simulink model "elec_switching_power_supply"  (R2016a)
settings: Solver=ode23t  StartTime=0.0  StopTime=0.006  RelTol=1e-3
PostLoadFcn:
  | controller_choice=1; % Variant selection variable
InitFcn:
  | if ~exist('T_junction1','var')
  |   T_junction1 = 404.79;
  | end
  | if ~exist('T_junction2','var')
  |   T_junction2 = 384.83;
  | end
libraries: fl_lib x11, elec_lib x7, nesl_utility x3, simulink x1
CloseFcn:
  | try close(h1_elec_switching_power_supply), end
  | try close(h2_elec_switching_power_supply), end
  | try clear elec_sps_log tout controller_choice, end
Description:
  | Synchronous Buck Converter
  | 
  | This example shows how to model a switching power supply that converts a 30V DC
  | supply into a regulated 15V DC supply. The model can be used to both size the
  | inductance L and smoothing capacitor C, as well as to design the feedback
  | controller. By selecting between continuous, discrete and fixed-point controllers, the
  | impact of discretization and using limited numerical precision can be explored.
  | 
  | Modeling the switching devices as MOSFETs rather than ideal switches ensures that
  | device on-resistances are correctly represented. The model also captures the
  | switch-on/switch-off timing of the devices, this depending primarily on the gate
  | capacitance values and the PWM driver output resistance.
  | 
  | If you have Simscape(TM) Power Systems(TM), see example model
  | power_switching_power_supply for an abstracted version of this model that
  | uses ideal switching to give faster simulation times. The model here can be used to
  | determine the on-resistance values required for the ideal switches, plus timing
  | offsets if necessary. Using the ideal switching approach of Simscape(TM) Power Systems
  | can be used to simulate more complex power converters.
  | 
  | Workspace variables T_junction1 and T_junction2 are used to define the
  | temperatures at which the two MOSFETs are simulated. Companion models
  | elec_switching_power_supply_thermal and
  | elec_switching_power_supply_thermal_only are used to determine these
  | temperatures.
  | 
  | 
  | 
  | 
  | 
  | 
  | Copyright 2008-2016 The MathWorks, Inc.
settings Model: FPTRunName=Active  Creator=MathWorks  LastModifiedBy=tmax4
settings DataIOCC: SaveFormat=Array  SignalLoggingSaveFormat=ModelDataLogs  SaveOutput=off  SignalLogging=off  DSMLogging=off  SignalLoggingName=sigsOut
settings OptimizationCC: BooleanDataType=off  ExpressionDepthLimit=2147483647  InitFltsAndDblsToZero=on  OptimizeModelRefInitCode=on  LifeSpan=1
settings DebuggingCC: SaveWithParameterizedLinksMsg=none  UnderspecifiedInitializationDetection=Classic  MergeDetectMultiDrivingBlocksExec=none  SignalResolutionControl=TryResolveAllWithWarning  MultiTaskDSMMsg=warning  MultiTaskCondExecSysMsg=none  IntegerOverflowMsg=none  ParameterPrecisionLossMsg=none  FcnCallInpInsideContextMsg=UseLocalSettings  AllowSymbolicDim=off  StateNameClashWarn=warning  IntegerSaturationMsg=none
settings HardwareCC: ProdBitPerPointer=32  ProdLargestAtomicFloat=None  ProdIntDivRoundTo=Undefined  ProdEndianess=Unspecified  ProdWordSize=32  ProdHWDeviceType=32-bit Generic
settings ModelReferenceCC: PropagateSignalLabelsOutOfModel=off
settings RTWCC: SystemTargetFile=ert.tlc  TemplateMakefile=ert_default_tmf  Description=Real-Time Workshop Embedded Coder (no auto configuration)  GenerateReport=on  IncludeHyperlinkInReport=on  LaunchReport=on  CreateSILPILBlock=SIL
settings CodeAppCC: IgnoreCustomStorageClasses=off  CustomSymbolStrType=$N$R$M  InternalIdentifier=Classic
settings ERTTargetCC: TargetFcnLib=ansi_tfl_tmw.mat  GenerateSampleERTMain=on  ERTCustomFileTemplate=example_file_process.tlc  ConvertIfToSwitch=off  SuppressUnreachableDefaultCases=off
settings ConfigComp: CovModelRefEnable=Off  CovSFcnEnable=off
settings SimscapeCC: SimscapeLogType=all  SimscapeLogName=elec_sps_log  SimscapeLogLimitData=off  SimscapeLogDataHistory=50000

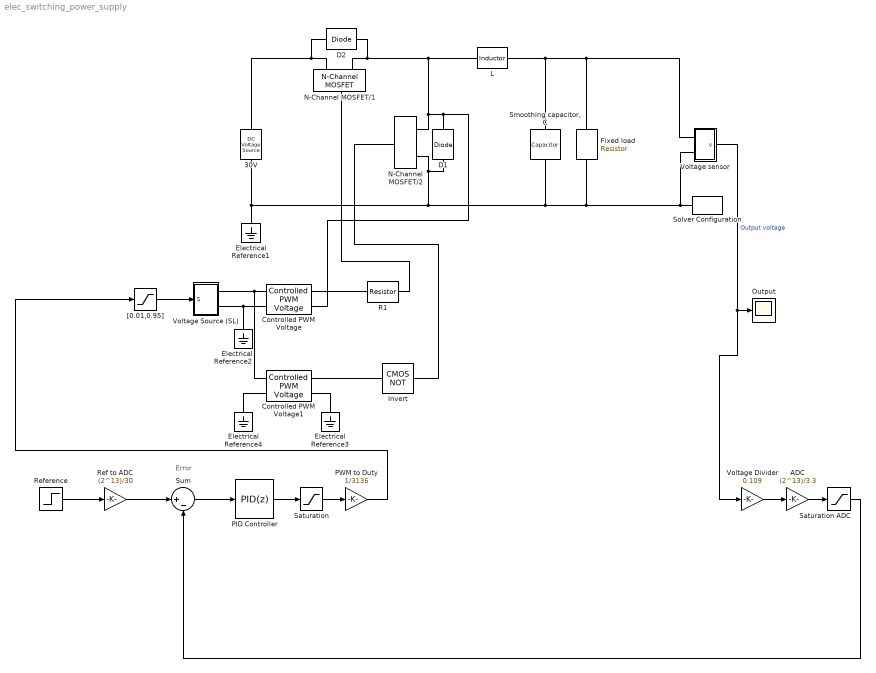
== system elec_switching_power_supply ==
  note: Error
  30V : fl_lib/Electrical/Electrical Sources/DC Voltage Source  v0=30 V
  ADC : Gain  Gain=(2^13)/3.3  OutDataTypeStr=uint16
  Controlled PWM Voltage : elec_lib/Actuators & Drivers/Drivers/Controlled PWM Voltage  F=50 kHz  TD=0 s  pulse_width_offset=0 s  Vmin=0 V  Vmax=1 V  Vm=30 V  pwm_or_av=1  event_type=1  sample_time=1e-6 s
  Controlled PWM Voltage1 : elec_lib/Actuators & Drivers/Drivers/Controlled PWM Voltage  F=50 kHz  TD=0 s  pulse_width_offset=0 s  Vmin=0 V  Vmax=1 V  Vm=30 V  pwm_or_av=1  event_type=1  sample_time=1e-6 s
  D1 : elec_lib/Semiconductor Devices/Diode  ModelType=3  Vf=0.6 V  Ron=0.3 Ohm  Goff=1e-8 S  Rz=0.3 Ohm  Vz=50 V  C_PWL=5 pF  prmExp=1  I12=[ 0.25 5 ] A  V12=[ 0.7 0.8 ] V  I1=0.07 A  V1=0.7 V  RS=0.01 Ohm  IS=1e-14 A  Tmeas=25 degC  ec=1  BV=Inf V  C_param=1  CJ0=100 pF  VJ=1 V  Mgrad=0.5  Vvec=[ 0.1 10 100 ] V  Cvec=[ 3.5 1 0.4 ] pF  FC=0.5  Q_param=1  Irrm=-7.15 A  iF=4 A  didt=-750 A/us  trr=115 ns  TT=50 ns  tau=100 ns  T_param=1  IS_T2=1.25e-7 A  I1_T2=0.245 A  V1_T2=0.5 V  Tmeas2=125 degC  EG_param=1  EG=1.11 eV  XTI_param=1  XTI=3  dBVdT=0 V/K  Tdevice=25 degC  Rth=[ 0 10 ] K/W  thermal_mass_parameterization=1  thermal_mass=[ 0 1 ] J/K  thermal_time_constant=[ 0 10 ] s  thermal_mass_initial_temperatures=[ 25 25 ] degC
  D2 : elec_lib/Semiconductor Devices/Diode  ModelType=3  Vf=0.6 V  Ron=0.3 Ohm  Goff=1e-8 S  Rz=0.3 Ohm  Vz=50 V  C_PWL=5 pF  prmExp=1  I12=[ 0.25 5 ] A  V12=[ 0.7 0.8 ] V  I1=0.07 A  V1=0.7 V  RS=0.01 Ohm  IS=1e-14 A  Tmeas=25 degC  ec=1  BV=Inf V  C_param=1  CJ0=100 pF  VJ=1 V  Mgrad=0.5  Vvec=[ 0.1 10 100 ] V  Cvec=[ 3.5 1 0.4 ] pF  FC=0.5  Q_param=1  Irrm=-7.15 A  iF=4 A  didt=-750 A/us  trr=115 ns  TT=50 ns  tau=100 ns  T_param=1  IS_T2=1.25e-7 A  I1_T2=0.245 A  V1_T2=0.5 V  Tmeas2=125 degC  EG_param=1  EG=1.11 eV  XTI_param=1  XTI=3  dBVdT=0 V/K  Tdevice=25 degC  Rth=[ 0 10 ] K/W  thermal_mass_parameterization=1  thermal_mass=[ 0 1 ] J/K  thermal_time_constant=[ 0 10 ] s  thermal_mass_initial_temperatures=[ 25 25 ] degC
  Electrical Reference{1..4} (4 alike) : fl_lib/Electrical/Electrical Elements/Electrical Reference
  Fixed load : fl_lib/Electrical/Electrical Elements/Resistor  R=10 Ohm  i_specify=off  i_priority=High  i=0 A  v_specify=off  v_priority=High  v=0 V
  Invert : elec_lib/Integrated Circuits/Logic/CMOS NOT  V_IL=10 V  V_IH=20 V  C_IN=0 pF  output_type=1  V_OL=0 V  V_OH=30 V  V_CC=5 V  V_meas=5 V  R_OUT=100 Ohm  R_OH=[ 25 250 ] Ohm  I_OH=63 mA  R_OL=[ 30 800 ] Ohm  I_OL=-45 mA  Delay=0 s  Ron=5 Ohm  Vf=0.6 V  output_state=1
  L : fl_lib/Electrical/Electrical Elements/Inductor  l=100e-6 H  r=118e-3 Ohm  g=0 1/Ohm  i_specify=off  i_priority=High  i=0 A  v_specify=off  v_priority=High  v=0 V  i_L_specify=on  i_L_priority=High  i_L=0 A
  N-Channel MOSFET/1 : elec_lib/Semiconductor Devices/N-Channel MOSFET  parameterization=1  prmDatasheet=2  prmEquCoeff=1  Beta=5 A/V^2  Rds=12.6e-3 Ohm  Id=15 A  Vgs=10 V  Vth=3 V  lam=0 1/V  Tmeas=25 degC  RS=6e-3 Ohm  RD=6e-3 Ohm  C_param=1  C_GS=270 pF  C_GD=80 pF  C_DS=0 pF  C_iss=1220 pF  C_rss=95 pF  C_oss=169 pF  C_GS_vec=[ 270 300 290 280 295 255 ] pF  C_GD_vec=[ 450 400 300 190 95 55 ] pF  C_DS_vec=[ 450 410 390 230 175 115 ] pF  C_iss_vec=[ 720 700 590 470 390 310 ] pF  C_rss_vec=[ 450 400 300 190 95 55 ] pF  C_oss_vec=[ 900 810 690 420 270 170 ] pF  C_Vds_vec=[ 0.1 0.3 1 3 10 30 ] V  charge_linearity_param=1  C_OX=200 pF  V_C_OX=-0.5 V  dVth_dT=-6 mV/K  Rds_T2=0.2 Ohm  Tmeas2=125 degC  BEXDatasheet=-1.5  BEXEquCoeff=-1.5  TdeviceDatasheet=30 degC  TdeviceEquCoeff=25 degC  Rth=[ 20 1 ] K/W  thermal_mass_parameterization=2  thermal_mass=[ 0.3 2 ] J/K  thermal_time_constant=[ 1 10 ] s  thermal_mass_initial_temperatures=[ 300 300 ] K
  N-Channel MOSFET/2 : elec_lib/Semiconductor Devices/N-Channel MOSFET  parameterization=1  prmDatasheet=2  prmEquCoeff=1  Beta=5 A/V^2  Rds=12.6e-3 Ohm  Id=15 A  Vgs=10 V  Vth=3 V  lam=0 1/V  Tmeas=25 degC  RS=6e-3 Ohm  RD=6e-3 Ohm  C_param=1  C_GS=270 pF  C_GD=80 pF  C_DS=0 pF  C_iss=1220 pF  C_rss=95 pF  C_oss=169 pF  C_GS_vec=[ 270 300 290 280 295 255 ] pF  C_GD_vec=[ 450 400 300 190 95 55 ] pF  C_DS_vec=[ 450 410 390 230 175 115 ] pF  C_iss_vec=[ 720 700 590 470 390 310 ] pF  C_rss_vec=[ 450 400 300 190 95 55 ] pF  C_oss_vec=[ 900 810 690 420 270 170 ] pF  C_Vds_vec=[ 0.1 0.3 1 3 10 30 ] V  charge_linearity_param=1  C_OX=200 pF  V_C_OX=-0.5 V  dVth_dT=-6 mV/K  Rds_T2=0.2 Ohm  Tmeas2=125 degC  BEXDatasheet=-1.5  BEXEquCoeff=-1.5  TdeviceDatasheet=30 degC  TdeviceEquCoeff=25 degC  Rth=[ 20 1 ] K/W  thermal_mass_parameterization=2  thermal_mass=[ 0.3 2 ] J/K  thermal_time_constant=[ 1 10 ] s  thermal_mass_initial_temperatures=[ 300 300 ] K
  Output : Scope
  PID Controller : simulink/Continuous/PID Controller  Controller=PID  TimeDomain=Discrete-time  SampleTime=6.66e-6  IntegratorMethod=Trapezoidal  FilterMethod=Forward Euler  Form=Parallel  UseFilter=off  ControllerParametersSource=internal  P=5  I=40000  D=0.000006  N=0.009092182911359  InitialConditionSource=internal  InitialConditionForIntegrator=0  InitialConditionForFilter=0  ExternalReset=none  LimitOutput=off  UpperSaturationLimit=inf  LowerSaturationLimit=-inf  LinearizeAsGain=on  AntiWindupMode=none  Kb=1  TrackingMode=off  Kt=1  PParamMin=[]  PParamMax=[]  PParamDataTypeStr=double  IParamMin=[]  IParamMax=[]  IParamDataTypeStr=double  DParamMin=[]  DParamMax=[]  DParamDataTypeStr=double  NParamMin=[]  NParamMax=[]  KbParamMin=[]  KbParamMax=[]  KtParamMin=[]  KtParamMax=[]  POutMin=[]  POutMax=[]  POutDataTypeStr=double  PGainOutDataTypeStr=double  PProdOutDataTypeStr=double  IOutMin=[]  IOutMax=[]  IOutDataTypeStr=double  IGainOutDataTypeStr=double  IProdOutDataTypeStr=double  DOutMin=[]  DOutMax=[]  DOutDataTypeStr=double  DGainOutDataTypeStr=double  DProdOutDataTypeStr=double  NOutMin=[]  NOutMax=[]  KbOutMin=[]  KbOutMax=[]  KtOutMin=[]  KtOutMax=[]  IntegratorOutMin=[]  IntegratorOutMax=[]  IntegratorOutDataTypeStr=double  FilterOutMin=[]  FilterOutMax=[]  SumOutMin=[]  SumOutMax=[]  SumOutDataTypeStr=double  SumI1OutMin=[]  SumI1OutMax=[]  SumI2OutMin=[]  SumI2OutMax=[]  SumI3OutMin=[]  SumI3OutMax=[]  SumDOutMin=[]  SumDOutMax=[]  SumAccumDataTypeStr=double  SaturationOutMin=[]  SaturationOutMax=[]  IntegratorContinuousStateAttributes=''  IntegratorStateMustResolveToSignalObject=off  IntegratorRTWStateStorageClass=Auto  FilterContinuousStateAttributes=''  FilterStateMustResolveToSignalObject=off  FilterRTWStateStorageClass=Auto  DifferentiatorICPrevScaledInput=0  DifferentiatorOutMin=[]  DifferentiatorOutMax=[]  DifferentiatorOutDataTypeStr=double
  PWM to Duty : Gain  Gain=1/3136  OutDataTypeStr=double
  R1 : fl_lib/Electrical/Electrical Elements/Resistor  R=5 Ohm  i_specify=off  i_priority=High  i=0 A  v_specify=off  v_priority=High  v=0 V
  Ref to ADC : Gain  Gain=(2^13)/30  OutDataTypeStr=uint16
  Reference : Step  Time=0  After=5  SampleTime=0
  Saturation : Saturate  UpperLimit=2822  LowerLimit=62  OutDataTypeStr=uint16
  Saturation ADC : Saturate  UpperLimit=2^13  LowerLimit=0  OutDataTypeStr=uint16
  "Smoothing capacitor, C" : fl_lib/Electrical/Electrical Elements/Capacitor  c=470 uF  r=0.35 Ohm  g=0 1/Ohm  i_specify=off  i_priority=High  i=0 A  v_specify=off  v_priority=High  v=0 V  vc_specify=on  vc_priority=High  vc=0 V
  Solver Configuration : nesl_utility/Solver Configuration  PhysicalDomain=network_engine_domain  SubClassName=solver  LeftPortType=input  RightPortType=generic  Accelerate=off  Tones=[]  Harmonics=[]  SimulateNoise=off  Profile=off  UseLocalSampling=off  EnableSwitchedLinearOptims=on  FrequencyDomain=off  UseCCode=off  RelTol=0.001  AbsTol=1e-06  MinStep=1e-09  ToWorkspace=off  RevertToSquareIcSolve=off  NumHomotopyIterations=100  PhasorMode=off  PhasorModeNumHarmonics=1  OverrideAbsTol=off  DoDC=off  ResidualTolerance=1e-9  UseLocalSolver=off  LocalSolverChoice=NE_BACKWARD_EULER_ADVANCER  LocalSolverSampleTime=1e-7  DoFixedCost=off  MaxNonlinIter=12  MaxModeIter=2  LinearAlgebra=Sparse  DelaysMemoryBudget=1024  AutomaticFiltering=on  FilteringTimeConstant=0.001
  Sum : Sum  Inputs=|+-  OutDataTypeStr=int16
  Voltage Source (SL) : Subsystem
      settings: CopyFcn=set_param(gcb,'LinkStatus','none')
  Voltage sensor : Subsystem
      settings: CopyFcn=set_param(gcb,'LinkStatus','none')
  Voltage Divider : Gain  Gain=0.109  OutDataTypeStr=double
  "[0.01,0.95]" : Saturate  UpperLimit=0.95  LowerLimit=.01
  wires:
  "[0.01,0.95]"/1 -> Voltage Source (SL)/1(S)
  Reference/1 -> Ref to ADC/1
  Sum/1 -> PID Controller/1
  Ref to ADC/1 -> Sum/1
  Saturation ADC/1 -> Sum/2
  PID Controller/1 -> Saturation/1
  Saturation/1 -> PWM to Duty/1
  Voltage Divider/1 -> ADC/1
  ADC/1 -> Saturation ADC/1
  PWM to Duty/1 -> "[0.01,0.95]"/1
  Voltage sensor/1(v) -> Output/1, Voltage Divider/1  "Output voltage"
  connections:
  N-Channel MOSFET/1/RConn2 -- L/RConn1 -- Controlled PWM Voltage/RConn2 -- D1/RConn1 -- N-Channel MOSFET/2/RConn1 -- D2/LConn1
  Voltage sensor/LConn1 -- L/LConn1 -- "Smoothing capacitor, C"/LConn1 -- Fixed load/LConn1
  N-Channel MOSFET/2/RConn2 -- D1/LConn1 -- Voltage sensor/LConn2 -- Solver Configuration/RConn1 -- Fixed load/RConn1 -- "Smoothing capacitor, C"/RConn1 -- 30V/RConn1 -- Electrical Reference1/LConn1
  R1/LConn1 -- N-Channel MOSFET/1/LConn1
  Invert/RConn1 -- N-Channel MOSFET/2/LConn1
  N-Channel MOSFET/1/RConn1 -- 30V/LConn1 -- D2/RConn1
  Controlled PWM Voltage/LConn1 -- Voltage Source (SL)/RConn1 -- Controlled PWM Voltage1/LConn1
  Electrical Reference2/LConn1 -- Voltage Source (SL)/RConn2 -- Controlled PWM Voltage/LConn2
  Controlled PWM Voltage1/LConn2 -- Electrical Reference4/LConn1
  Electrical Reference3/LConn1 -- Controlled PWM Voltage1/RConn2
  Controlled PWM Voltage1/RConn1 -- Invert/LConn1
  Controlled PWM Voltage/RConn1 -- R1/RConn1

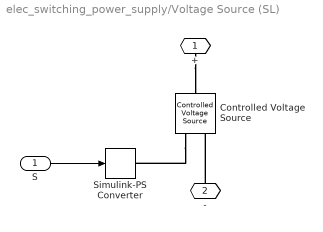
== system elec_switching_power_supply/Voltage Source (SL) ==
  S : Inport
  Controlled Voltage Source : fl_lib/Electrical/Electrical Sources/Controlled Voltage Source
  Simulink-PS Converter : nesl_utility/Simulink-PS Converter  PhysicalDomain=network_engine_domain  SubClassName=ps_input  LeftPortType=input  RightPortType=output  PseudoPeriodic=off  Frequencies=[]  NoiseDistribution=none  NoiseParameters=[]  Unit=V  AffineConversion=off  InputFiltering=off  SimscapeFilterOrder=1  InputFilterTimeConstant=.001  UdotUserProvided=0
  + : PMIOPort  Port=1  Side=Right
  - : PMIOPort  Port=2  Side=Right
  wires:
  S/1 -> Simulink-PS Converter/1
  connections:
  +/RConn1 -- Controlled Voltage Source/LConn1
  -/RConn1 -- Controlled Voltage Source/RConn2
  Controlled Voltage Source/RConn1 -- Simulink-PS Converter/RConn1

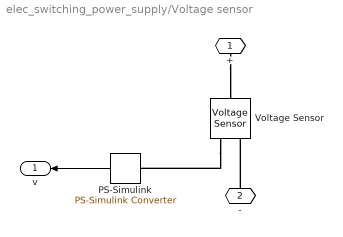
== system elec_switching_power_supply/Voltage sensor ==
  PS-Simulink : nesl_utility/PS-Simulink Converter  PhysicalDomain=network_engine_domain  SubClassName=ps_output  LeftPortType=input  RightPortType=output  PseudoPeriodic=off  Frequencies=[]  Unit=V  AffineConversion=off
  Voltage Sensor : fl_lib/Electrical/Electrical Sensors/Voltage Sensor
  + : PMIOPort  Port=1  Side=Left
  - : PMIOPort  Port=2  Side=Left
  v : Outport
  wires:
  PS-Simulink/1 -> v/1
  connections:
  Voltage Sensor/RConn1 -- PS-Simulink/LConn1
  +/RConn1 -- Voltage Sensor/LConn1
  -/RConn1 -- Voltage Sensor/RConn2
